simulink model "data_acquisition_file_slider_pre_defined_inputs"  (R2019b)
settings: Solver=VariableStepAuto  StartTime=0.0  StopTime=30  RelTol=1e-3
undefined symbols (not defined in the file or in its folder): sigbuilder_block
settings Model: EnablePacing=on  Creator=mandl  LastModifiedBy=mandl

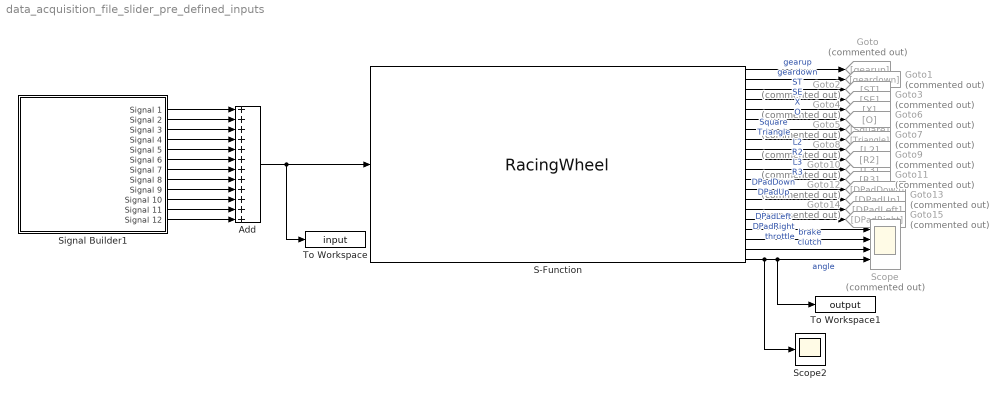
== system data_acquisition_file_slider_pre_defined_inputs ==
  Add : Sum  Inputs=++++++++++++
  Goto : Goto  Commented=on  GotoTag=gearup
  Goto1 : Goto  Commented=on  GotoTag=geardown
  Goto10 : Goto  Commented=on  GotoTag=L3
  Goto11 : Goto  Commented=on  GotoTag=R3
  Goto12 : Goto  Commented=on  GotoTag=DPadDown
  Goto13 : Goto  Commented=on  GotoTag=DPadUp
  Goto14 : Goto  Commented=on  GotoTag=DPadLeft
  Goto15 : Goto  Commented=on  GotoTag=DPadRight
  Goto2 : Goto  Commented=on  GotoTag=ST
  Goto3 : Goto  Commented=on  GotoTag=SE
  Goto4 : Goto  Commented=on  GotoTag=X
  Goto5 : Goto  Commented=on  GotoTag=Square
  Goto6 : Goto  Commented=on  GotoTag=O
  Goto7 : Goto  Commented=on  GotoTag=Triangle
  Goto8 : Goto  Commented=on  GotoTag=L2
  Goto9 : Goto  Commented=on  GotoTag=R2
  S-Function : S-Function  FunctionName=RacingWheel  Parameters=Ts_FF  SFunctionModules=RacingWheel_wrapper  SFunctionDeploymentMode=off  EnableBusSupport=off  mask(Racing Wheel with Force Feedback){Ts_FF=0.01}
      mask prompts: Ts_FF "Constant Force-Feedback Sample Time"
      mask help: Interacts with the windows gaming API from UWP. The force feedback effect is constant over the user defined sampling time below.
      mask init:
      | val = [[.9  0.75 0.75 1 1 .9 .9 1]',[1 1 0.75 0.75 .9 .9 1 .9]'];try , sys = get_param(gcb,'SfunBuilderFcnName');if isempty(sys), sys = get_param(gcb,'FunctionName'); end,catch, sys = get_param(gcb,'FunctionName'); end
      mask Display:
      | plot(val(:,1),val(:,2)),disp(sys),
      | image('icon.png'),
      | port_label('input',1,'FF'),
      | port_label('output',1,'gearup'),
      | port_label('output',2,'geardown'),
      | port_label('output',3,'ST'),
      | port_label('output',4,'SE'),
      | port_label('output',5,'X'),
      | port_label('output',6,'O'),
      | port_label('output',7,'Square'),
      | port_label('output',8,'Triangle'),
      | port_label('output',9,'L2'),
      | port_label('output',10,'R2'),
      | port_label('output',11,'L3'),
      | port_label('output',12,'R3'),
      | port_label('output',13,'DPadDown'),
      | port_label('output',14,'DPadUp'),
      | port_label('output',15,'DPadLeft'),
      | port_label('output',16,'DPadRight'),
      | port_label('output',17,'throttle'),
      | port_label('output',18,'brake'),
      | port_label('output',19,'clutch'),
      | port_label('output',20,'angle')
  Scope : Scope  Commented=on  NumInputPorts=4
  Scope2 : Scope
  Signal Builder1 : Subsystem  Tag=STV Subsys  LoadFcn=sigbuilder_block('load');  StartFcn=sigbuilder_block('start');  StopFcn=sigbuilder_block('stop');  ClipboardFcn=sigbuilder_block('clipboard');  mask(Sigbuilder block){tuvar=[0:10]}
      mask help: Simulink:masks:SigbuilderBlock_MD
      mask init:
      | if ~strcmp(get_param(bdroot(gcbh),'SimulationStatus'),'stopped') tuvar = sigbuilder_block('maskInit'); end
      settings: CopyFcn=sigbuilder_block('copy');  DeleteFcn=sigbuilder_block('delete');  ModelCloseFcn=sigbuilder_block('modelClose');  PreSaveFcn=sigbuilder_block('preSave');  PauseFcn=sigbuilder_block('pause');  ContinueFcn=sigbuilder_block('continue');  NameChangeFcn=sigbuilder_block('namechange');  OpenFcn=sigbuilder_block('open',[0.75 30.75 958.5 985.5 ]);  CloseFcn=sigbuilder_block('close');
      mask Display: plot(0, 0, 100, 100,[2, 2, 32, 32, 2], [68, 8, 8, 68, 68],[32, 2], [38, 38], [32, 19, 2],[53, 60, 44], [32, 17, 17, 2],[16, 16, 31, 31]);txt = getActiveGroup(gcbh);text(2, 100, txt,'verticalAlignment', 'top');
  To Workspace : ToWorkspace  VariableName=input  SaveFormat=Structure With Time  SampleTime=0.01
  To Workspace1 : ToWorkspace  VariableName=output  SaveFormat=Structure With Time  SampleTime=0.01
  wires:
  S-Function/19 -> Scope/3  "clutch"
  S-Function/18 -> Scope/2  "brake"
  S-Function/17 -> Scope/1  "throttle"
  S-Function/1 -> Goto/1  "gearup"
  S-Function/2 -> Goto1/1  "geardown"
  S-Function/3 -> Goto2/1  "ST"
  S-Function/4 -> Goto3/1  "SE"
  S-Function/5 -> Goto4/1  "X"
  S-Function/6 -> Goto6/1  "O"
  S-Function/7 -> Goto5/1  "Square"
  S-Function/8 -> Goto7/1  "Triangle"
  S-Function/9 -> Goto8/1  "L2"
  S-Function/10 -> Goto9/1  "R2"
  S-Function/11 -> Goto10/1  "L3"
  S-Function/12 -> Goto11/1  "R3"
  S-Function/13 -> Goto12/1  "DPadDown"
  S-Function/14 -> Goto13/1  "DPadUp"
  S-Function/15 -> Goto14/1  "DPadLeft"
  S-Function/16 -> Goto15/1  "DPadRight"
  Signal Builder1/1(Signal 1) -> Add/1
  Signal Builder1/2(Signal 2) -> Add/2
  Signal Builder1/3(Signal 3) -> Add/3
  Signal Builder1/4(Signal 4) -> Add/4
  Signal Builder1/5(Signal 5) -> Add/5
  Signal Builder1/6(Signal 6) -> Add/6
  Signal Builder1/7(Signal 7) -> Add/7
  Signal Builder1/8(Signal 8) -> Add/8
  Signal Builder1/9(Signal 9) -> Add/9
  Signal Builder1/10(Signal 10) -> Add/10
  Signal Builder1/11(Signal 11) -> Add/11
  Signal Builder1/12(Signal 12) -> Add/12
  S-Function/20 -> Scope2/1, To Workspace1/1, Scope/4  "angle"
  Add/1 -> To Workspace/1, S-Function/1

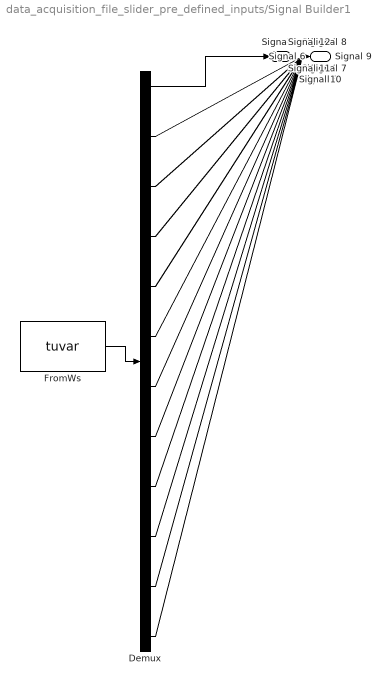
== system data_acquisition_file_slider_pre_defined_inputs/Signal Builder1 ==
  Demux : Demux  Tag=STV Demux  Outputs=12
  FromWs : FromWorkspace  Tag=STV FromWs  VariableName=tuvar  SampleTime=0
      SigBuilderData=|
      | common.afterFinalStr = 'Extrapolate'
      | common.sampleTime = 0
      | dataSet.timeRange = [0 30]
      | dataSet.name = 'Group 1'
      | sbobj.Groups.Name = 'Group 1'
      | sbobj.Groups.Signals(1).Name = 'Signal 1'
      | sbobj.Groups.Signals(1).XData = [0 0.5 0.5 0.51 0.51 30]
      | sbobj.Groups.Signals(1).YData = [0 0 0.8 0.8 0 0]
      | sbobj.Groups.Signals(2).Name = 'Signal 2'
      | sbobj.Groups.Signals(2).XData = [0 1 1 1.5 1.5 30]
      | sbobj.Groups.Signals(2).YData = [0 0 0.35 0.35 0 0]
      | sbobj.Groups.Signals(3).Name = 'Signal 3'
      | sbobj.Groups.Signals(3).XData = [0 3 3 3.8 3.8 30]
      | sbobj.Groups.Signals(3).YData = [0 0 -0.5 -0.5 0 0]
      | sbobj.Groups.Signals(4).Name = 'Signal 4'
      | sbobj.Groups.Signals(4).XData = [0 5 5 5.8 5.8 30]
      | sbobj.Groups.Signals(4).YData = [0 0 0.25 0.25 0 0]
      | sbobj.Groups.Signals(5).Name = 'Signal 5'
      | sbobj.Groups.Signals(5).XData = [0 7 7 7.5 7.5 30]
      | sbobj.Groups.Signals(5).YData = [0 0 -0.2 -0.2 0 0]
      | sbobj.Groups.Signals(6).Name = 'Signal 6'
      | sbobj.Groups.Signals(6).XData = [0 9 9 10 10 30]
      | sbobj.Groups.Signals(6).YData = [0 0 -0.18 -0.18 0 0]
      | sbobj.Groups.Signals(7).Name = 'Signal 7'
      | sbobj.Groups.Signals(7).XData = [0 13 13 14 14 30]
      | sbobj.Groups.Signals(7).YData = [0 0 0.19 0.19 0 0]
      | sbobj.Groups.Signals(8).Name = 'Signal 8'
      | sbobj.Groups.Signals(8).XData = [0 17 17 17.1 17.1 30]
      | sbobj.Groups.Signals(8).YData = [0 0 -1 -1 0 0]
      | sbobj.Groups.Signals(9).Name = 'Signal 9'
      | sbobj.Groups.Signals(9).XData = [0 20 20 20.2 20.2 30]
      | sbobj.Groups.Signals(9).YData = [0 0 -0.5 -0.5 0 0]
      | sbobj.Groups.Signals(10).Name = 'Signal 10'
      | sbobj.Groups.Signals(10).XData = [0 22 22 22.2 22.2 30]
      | sbobj.Groups.Signals(10).YData = [0 0 0.5 0.5 0 0]
      | sbobj.Groups.Signals(11).Name = 'Signal 11'
      | sbobj.Groups.Signals(11).XData = [0 25 25 25.1 25.1 30]
      | sbobj.Groups.Signals(11).YData = [0 0 -1 -1 0 0]
      | sbobj.Groups.Signals(12).Name = 'Signal 12'
      | sbobj.Groups.Signals(12).XData = [0 27 27 27.1 27.1 30]
      | sbobj.Groups.Signals(12).YData = [0 0 1 1 0 0]
      | sbobj.Groups.TimeRange = [0 30]
  Signal 1 : Outport  Tag=STV Outport
  Signal 2 : Outport  Tag=STV Outport  Port=2
  Signal 3 : Outport  Tag=STV Outport  Port=3
  Signal 4 : Outport  Tag=STV Outport  Port=4
  Signal 5 : Outport  Tag=STV Outport  Port=5
  Signal 6 : Outport  Tag=STV Outport  Port=6
  Signal 7 : Outport  Tag=STV Outport  Port=7
  Signal 8 : Outport  Tag=STV Outport  Port=8
  Signal 9 : Outport  Tag=STV Outport  Port=9
  Signal 10 : Outport  Tag=STV Outport  Port=10
  Signal 11 : Outport  Tag=STV Outport  Port=11
  Signal 12 : Outport  Tag=STV Outport  Port=12
  wires:
  Demux/1 -> Signal 1/1
  FromWs/1 -> Demux/1
  Demux/2 -> Signal 2/1
  Demux/3 -> Signal 3/1
  Demux/4 -> Signal 4/1
  Demux/5 -> Signal 5/1
  Demux/6 -> Signal 6/1
  Demux/7 -> Signal 7/1
  Demux/8 -> Signal 8/1
  Demux/9 -> Signal 9/1
  Demux/10 -> Signal 10/1
  Demux/11 -> Signal 11/1
  Demux/12 -> Signal 12/1
